simulink subsystem "swing_planning"  (R2022b)
settings: Solver=VariableStepAuto  StartTime=0.0  StopTime=10.0  RelTol=1e-3
settings Model: Creator=LiAn  LastModifiedBy=LiAn

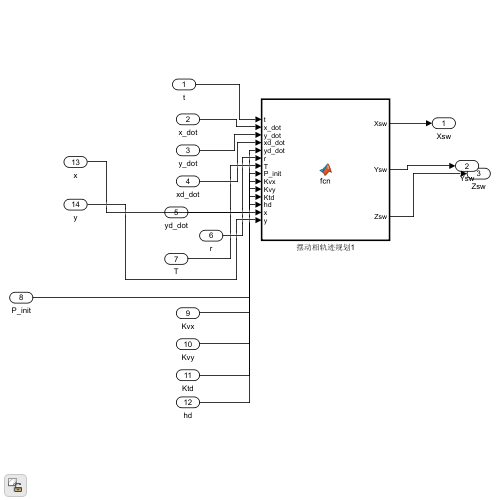
[thumbnail: Simulink's stored preview of the top-level diagram]
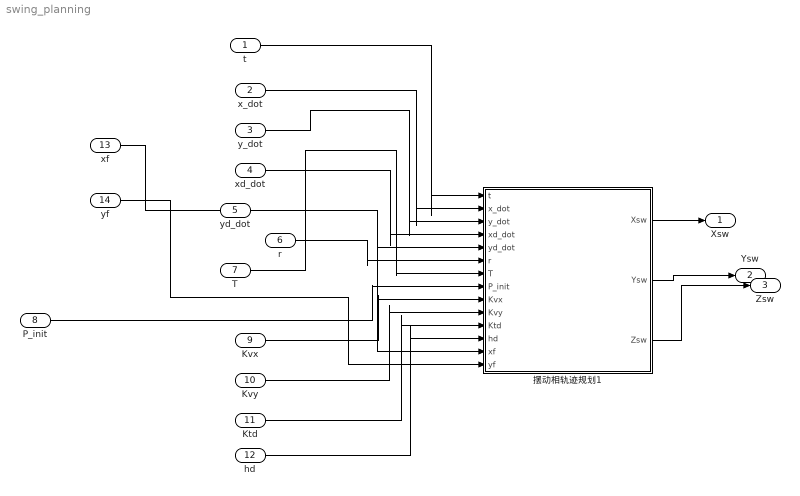
== system swing_planning ==
  t : Inport
  x_dot : Inport  Port=2
  y_dot : Inport  Port=3
  xd_dot : Inport  Port=4
  yd_dot : Inport  Port=5
  r : Inport  Port=6
  T : Inport  Port=7
  P_init : Inport  Port=8
  Kvx : Inport  Port=9
  Kvy : Inport  Port=10
  Ktd : Inport  Port=11
  hd : Inport  Port=12
  xf : Inport  Port=13
  yf : Inport  Port=14
  摆动相轨迹规划1 : MATLAB Function  TreatAsAtomicUnit=on
  Xsw : Outport
  Ysw : Outport  Port=2
  Zsw : Outport  Port=3
  wires:
  摆动相轨迹规划1/2(Ysw) -> Ysw/1
  r/1 -> 摆动相轨迹规划1/6(r)
  Kvx/1 -> 摆动相轨迹规划1/9(Kvx)
  摆动相轨迹规划1/3(Zsw) -> Zsw/1
  xf/1 -> 摆动相轨迹规划1/13(xf)
  摆动相轨迹规划1/1(Xsw) -> Xsw/1
  xd_dot/1 -> 摆动相轨迹规划1/4(xd_dot)
  t/1 -> 摆动相轨迹规划1/1(t)
  yf/1 -> 摆动相轨迹规划1/14(yf)
  Kvy/1 -> 摆动相轨迹规划1/10(Kvy)
  Ktd/1 -> 摆动相轨迹规划1/11(Ktd)
  P_init/1 -> 摆动相轨迹规划1/8(P_init)
  x_dot/1 -> 摆动相轨迹规划1/2(x_dot)
  y_dot/1 -> 摆动相轨迹规划1/3(y_dot)
  yd_dot/1 -> 摆动相轨迹规划1/5(yd_dot)
  hd/1 -> 摆动相轨迹规划1/12(hd)
  T/1 -> 摆动相轨迹规划1/7(T)

== matlab function swing_planning/摆动相轨迹规划1 ==
  data: t input; x_dot input; Xsw output; y_dot input; xd_dot input; yd_dot input; r input; T input; P_init input; Kvx input; Kvy input; Ktd input; hd input; Ysw output; Zsw output; xf input; yf input
function [Xsw,Ysw,Zsw] = fcn(t,x_dot,y_dot,xd_dot,yd_dot,r,T,P_init,Kvx,Kvy,Ktd,hd,xf,yf)

x_init = P_init(1);
y_init = P_init(2);
z_init = P_init(3);

Tsw = r*T;
Tst = T-Tsw;

if(t>Tsw)
    deta_t = t-Tsw;
    phi = 2*pi;
    Xsw = xf+x_init;
    Ysw = yf+y_init;
else
    deta_t=0;
    phi = 2*pi*t/Tsw;
    Xsw = xf*(phi-sin(phi))/(2*pi)+x_init;
    Ysw = yf*(phi-sin(phi))/(2*pi)+y_init;
end
 

Zsw = hd*(1-cos(phi))/2 + z_init - Ktd*(deta_t);
 
 
end
